simulink model "case_7_zero_relative_v_low_gap"  (R2025b)
settings: Solver=VariableStepAuto  StartTime=0.0  StopTime=5  RelTol=1e-3
settings Model: Creator=sanborkl  LastModifiedBy=admin

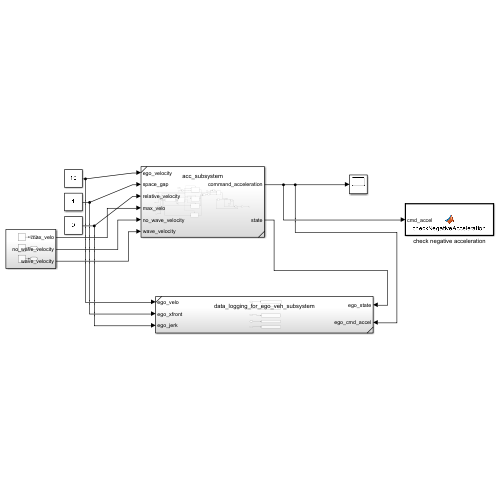
[thumbnail: Simulink's stored preview of the top-level diagram]
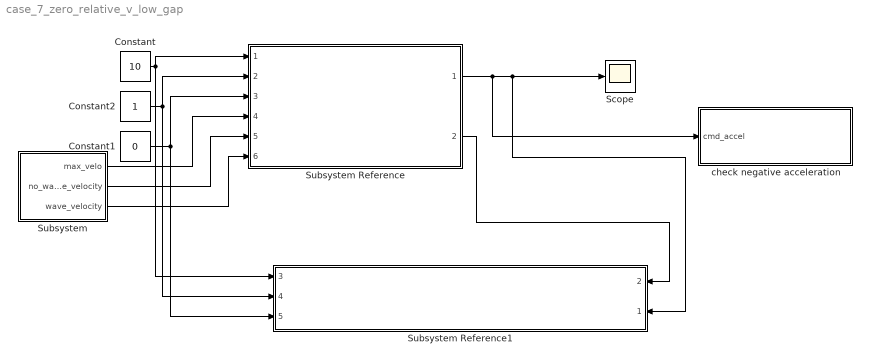
== system case_7_zero_relative_v_low_gap ==
  Constant : Constant  Value=10
  Constant1 : Constant  Value=0
  Constant2 : Constant
  Scope : Scope
      settings: ActiveDisplayYMinimum=-4.2230986039788005  ActiveDisplayYMaximum=-1.2078627872485264
  Subsystem : Subsystem
  Subsystem Reference : Subsystem  ReferencedSubsystem=acc_subsystem
  Subsystem Reference1 : Subsystem  ReferencedSubsystem=data_logging_for_ego_veh_subsystem
      settings: PortSchema="{\"entries\":[{\"content\":{\"sides\":[{\"content\":{\"connectorIds\":[\"In3\",\"In4\",\"In5\"]},\"type\":\"ConnectorPlacement.EquallySpacedRectSide\",\"uuid\":\"0b96bcaa-a470-46c9-9268-f4bd6b1035a8\"},{\"content\":{\"connectorIds\":[\"In2\",\"In1\"],\"side\":\"RIGHT\"},\"type\":\"ConnectorPlacement.EquallySpacedRectSide\",\"uuid\":\"8e49005a-1e53-4e76-b163-50df0eb9f2cc\"},{\"content\":{\"side\":\"TOP\"},\"type\":\"ConnectorPlacement.EquallySpacedRectSide\",\"uuid\":\"3ff4af65-efca-4a64-9b7f-f479498e89e2\"}]},\"type\":\"ConnectorPlacement.EquallySpacedConnector\",\"uuid\":\"f10caef7-9599-4d5c-a8fd-3eb49f6fcaa8\"}],\"packageUris\":[\"http://schema.mathworks.com/mf0/Connector/R2020b\"],\"version\":\"1.0\"}"
  check negative acceleration : MATLAB Function  TreatAsAtomicUnit=on
  wires:
  Constant1/1 -> Subsystem Reference1/5, Subsystem Reference/3
  Constant2/1 -> Subsystem Reference1/4, Subsystem Reference/2
  Subsystem Reference/1 -> check negative acceleration/1(cmd_accel), Subsystem Reference1/1, Scope/1
  Constant/1 -> Subsystem Reference1/3, Subsystem Reference/1
  Subsystem Reference/2 -> Subsystem Reference1/2
  Subsystem/2(no_wave_velocity) -> Subsystem Reference/5
  Subsystem/1(max_velo) -> Subsystem Reference/4
  Subsystem/3(wave_velocity) -> Subsystem Reference/6

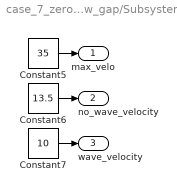
== system case_7_zero_relative_v_low_gap/Subsystem ==
  Constant5 : Constant  Value=35
  Constant6 : Constant  Value=13.5
  Constant7 : Constant  Value=10
  max_velo : Outport
  no_wave_velocity : Outport  Port=2
  wave_velocity : Outport  Port=3
  wires:
  Constant7/1 -> wave_velocity/1
  Constant6/1 -> no_wave_velocity/1
  Constant5/1 -> max_velo/1

== matlab function case_7_zero_relative_v_low_gap/check negative acceleration ==
  data: cmd_accel input
function checkNegativeAcceleration(cmd_accel)
%#codegen
coder.extrinsic('disp', 'sprintf');

if cmd_accel > 0
    msg = sprintf('Error: positive command acceleration: %.3f, should be 0 or negative', ...
                  cmd_accel);
    disp(msg);
end
end
